simulink model "Project_simulation_v2"  (R2022b)
settings: Solver=VariableStepAuto  StartTime=0.0  StopTime=15  RelTol=1e-3
libraries: spsDiodeLib x7, simulink x4, spsVoltageMeasurementLib x4, spsACVoltageSourceLib x3, spsCurrentMeasurementLib x3, spsMeanLib x3, spsRMSLib x2, spsDCMachineLib x1, spsDCVoltageSourceLib x1, spsIGBTLib x1, spsSeriesRLCBranchLib x1, sps_lib x1
settings Model: Creator=tunaa  LastModifiedBy=tunaa

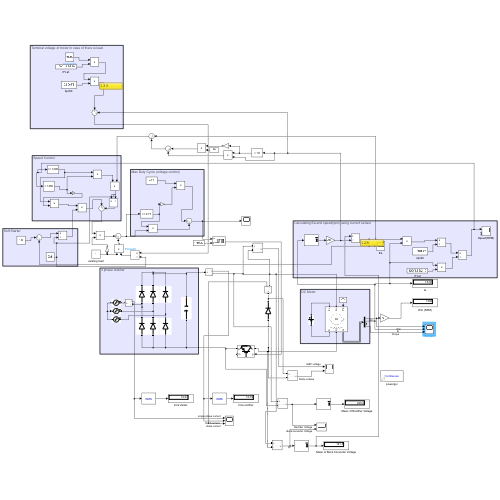
[thumbnail: Simulink's stored preview of the top-level diagram]
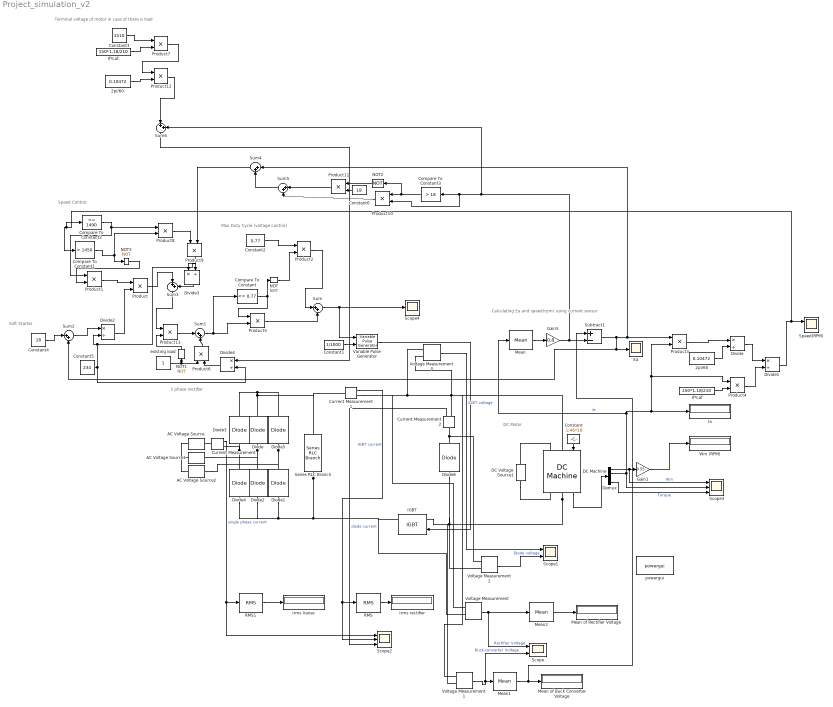
== system Project_simulation_v2 ==
  note: Speed Control
  note: DC Motor
  note: 3 phase rectifier
  note: Max Duty Cycle (voltage control)
  note: Calculating Ea and speed(rpm) using current sensor
  note: Soft Starter
  note: Terminal voltage of motor in case of there is load
  2pi/60 : Constant  Value=0.10472
  2pi/60. : Constant  Value=0.10472
  AC Voltage Source : spsACVoltageSourceLib/AC Voltage Source  Amplitude=136  Phase=0  Frequency=50  SampleTime=0  Measurements=None  BusType=swing  Pref=10e3  Qref=0  Qmin=-inf  Qmax=+inf
  AC Voltage Source1 : spsACVoltageSourceLib/AC Voltage Source  Amplitude=136  Phase=-120  Frequency=50  SampleTime=0  Measurements=None  BusType=swing  Pref=10e3  Qref=0  Qmin=-inf  Qmax=+inf
  AC Voltage Source2 : spsACVoltageSourceLib/AC Voltage Source  Amplitude=136  Phase=-240  Frequency=50  SampleTime=0  Measurements=None  BusType=swing  Pref=10e3  Qref=0  Qmin=-inf  Qmax=+inf
  Compare To Constant : simulink/Logic and Bit Operations/Compare To Constant  relop=<=  const=0.77  OutDataTypeStr=boolean
  Compare To Constant1 : simulink/Logic and Bit Operations/Compare To Constant  relop=>  const=1450  OutDataTypeStr=boolean
  Compare To Constant2 : simulink/Logic and Bit Operations/Compare To Constant  relop=<=  const=1490  OutDataTypeStr=boolean
  Compare To Constant3 : simulink/Logic and Bit Operations/Compare To Constant  relop=>  const=18  OutDataTypeStr=boolean
  Constant : Constant  Value=1.46*10
  Constant1 : Constant  Value=1/1000
  Constant2 : Constant  Value=0.77
  Constant3 : Constant  Value=1510
  Constant4 : Constant  Value=18
  Constant5 : Constant  Value=234
  Constant6 : Constant  Value=18
  Current Measurement : spsCurrentMeasurementLib/Current Measurement  PhasorSimulation=off  OutputType=Complex  PSBequivalent=0
  Current Measurement1 : spsCurrentMeasurementLib/Current Measurement  PhasorSimulation=off  OutputType=Complex  PSBequivalent=0
  Current Measurement2 : spsCurrentMeasurementLib/Current Measurement  PhasorSimulation=off  OutputType=Complex  PSBequivalent=0
  DC Machine : spsDCMachineLib/DC Machine  PresetModel=No  MechanicalLoad=Torque TL  FieldType=Wound  ShowDetailedParameters=on  MeasurementBus=off  RLa="[ 0.8  0.0125]"  RLf="[ 210  23]"  Laf=1.18  MachineConstant=Torque constant (N.m/A)  Ke=1.8  Kt=1.8  J=1  Bm=0  Tf=0  w0=157  Ifinit=0.714285714285714  TsPowergui=0  TsBlock=-1
  DC Voltage Source1 : spsDCVoltageSourceLib/DC Voltage Source  Amplitude=150  Measurements=None
  Demux : Demux
  Diode{,1..6} (7 alike) : spsDiodeLib/Diode  Ron=0.001  Lon=0  Vf=0.8  IC=0  UseSnubber=0  Rs=0  Cs=0  Measurements=off
  Divide{,1..4} (5 alike) : Product  Inputs=*/
  Ea : Scope
  Gain1 : Gain  Gain=9.55
  Gain5 : Gain  Gain=0.8
  IGBT : spsIGBTLib/IGBT  Ron=0.001  Lon=0  Vf=1  Tf=1e-6  Tt=2e-6  IC=0  Rs=1e5  Cs=inf  Measurements=on
  Ia : Display
  If*Laf : Constant  Value=150*1.18/210
  If*Laf. : Constant  Value=150*1.18/210
  Irms Variac : Display
  Irms rectifier : Display
  Mean : spsMeanLib/Mean  Freq=1000  Vinit=0  Ts=0
  Mean of Buck Converter Voltage : Display
  Mean of Rectifier Voltage : Display
  Mean1 : spsMeanLib/Mean  Freq=50  Vinit=0  Ts=0
  Mean2 : spsMeanLib/Mean  Freq=50  Vinit=0  Ts=0
  NOT{,1..3} (4 alike) : Logic  Operator=NOT  IconShape=distinctive  AllPortsSameDT=off  OutDataTypeStr=boolean
  Product{,1..13} (14 alike) : Product
  RMS : spsRMSLib/RMS  TrueRMS=on  Freq=50  RMSInit=0  Ts=0
  RMS1 : spsRMSLib/RMS  TrueRMS=on  Freq=50  RMSInit=0  Ts=0
  Scope : Scope  NumInputPorts=2
  Scope1 : Scope  NumInputPorts=2
  Scope2 : Scope  NumInputPorts=3
  Scope3 : Scope  NumInputPorts=3
  Scope4 : Scope
  Series RLC Branch : spsSeriesRLCBranchLib/Series RLC Branch  LConnTagsString=__new0  RConnTagsString=__new0  BranchType=C  Resistance=1  Inductance=1e-3  SetiL0=off  InitialCurrent=0  Capacitance=2*470e-6  Setx0=off  InitialVoltage=0  Measurements=None
  Speed(RPM) : Scope  NumInputPorts=2
  Subtract1 : Sum  Inputs=+-
  Sum{,1..6} (7 alike) : Sum  Inputs=|++
  Variable Pulse Generator : VariablePulseGenerator  AllowZeroPulseWidth=on  SampleTime=0.1
  Voltage Measurement{,1..3} (4 alike) : spsVoltageMeasurementLib/Voltage Measurement  PhasorSimulation=off  OutputType=Complex  PSBequivalent=0
  Wm (RPM) : Display
  existing load : Constant
  powergui : sps_lib/powergui  Priority=1  SimulationMode=Continuous  SampleTime=50e-6  frequency=60  Iterations=50  frequencyindice=50  Pbase=100e6  ErrMax=1e-4  UnitsV=kV  UnitsW=MW  buscounter=0  FunctionMessages=off  echomessages=off  EnableUseOfTLC=off  CurrentSourceSwitches=off  DisableSnubberDevices=off  DisableRonSwitches=off  DisableVfSwitches=off  DisplayEquations=off  AutomaticDiscreteSolvers=off  SolverType=Tustin/Backward Euler (TBE)  Interpol=off  ExternalGateDelay=off  methode=off  Ts=100  x0status=blocks  SPID=on  SwTol=0  HookPort=off  NonlinearTolerance=1e-4  nMaxIteration=100  ContinueOnMaxIteration=off  RestoreLinks=warning  ResistiveCurrentMeasurement=off  Frange=[0:2:500]  Ylog=off  Xlog=on  ShowGrid=off  save=off  variable=ZData  structure=0  ZoomFFT=off  StartTime=0.0  cycles=1  DisplayStyle=1  fundamental=60  FreqAxis=off  MaxFrequency=1000  frequencyindicesteady=1  RmsSteady=1  display=off
  wires:
  Current Measurement2/1 -> Scope2/3  "diode current"
  Subtract1/1 -> Sum2/2, Ea/1, Sum4/1, Product3/1
  Gain1/1 -> Wm (RPM)/1
  Demux/1 -> Scope3/1, Gain1/1  "Wm"
  Voltage Measurement3/1 -> Scope1/1  "IGBT voltage"
  Constant/1 -> DC Machine/1
  Constant2/1 -> Product2/1
  Demux/4 -> Scope3/3  "Torque"
  Product4/1 -> Divide1/2
  Constant5/1 -> Divide3/2, Divide2/2, Divide4/2
  Product2/1 -> Sum/1
  Constant4/1 -> Sum2/1
  Divide2/1 -> Product/2
  Current Measurement/1 -> Scope2/1, RMS1/1  "single phase current"
  Sum/1 -> Variable Pulse Generator/1, Scope4/1
  Product1/1 -> Product/1
  Compare To Constant/1 -> Product5/1, NOT/1
  NOT/1 -> Product2/2
  Divide/1 -> Divide1/1
  2pi/60/1 -> Divide/2
  Product5/1 -> Sum/2
  Product3/1 -> Divide/1
  Variable Pulse Generator/1 -> IGBT/1
  RMS/1 -> Irms rectifier/1
  Current Measurement1/1 -> Scope2/2, RMS/1  "IGBT current"
  Demux/2 -> Mean/1, Product4/1, Product3/2, Ia/1, Scope3/2  "Ia"
  RMS1/1 -> Irms Variac/1
  Sum2/1 -> Divide2/1
  Mean1/1 -> Subtract1/1, Mean of Buck Converter Voltage/1
  Voltage Measurement1/1 -> Scope/2, Mean1/1  "Buck-converter Voltage"
  Voltage Measurement/1 -> Scope/1, Mean2/1  "Rectifier Voltage"
  Constant1/1 -> Variable Pulse Generator/2
  DC Machine/1 -> Demux/1
  If*Laf/1 -> Product4/2
  Gain5/1 -> Sum6/2, Product10/2, Compare To Constant3/1, Subtract1/2
  Mean2/1 -> Mean of Rectifier Voltage/1
  Voltage Measurement2/1 -> Scope1/2  "Diode voltage"
  Mean/1 -> Gain5/1
  Compare To Constant1/1 -> NOT3/1, Product8/2
  NOT3/1 -> Product1/2
  Compare To Constant2/1 -> Product1/1, Product8/1
  Product8/1 -> Product9/1
  Product/1 -> Sum3/1
  Compare To Constant3/1 -> NOT2/1, Product10/1
  NOT2/1 -> Product11/1
  Constant6/1 -> Product11/2
  Product10/1 -> Sum5/2
  Product11/1 -> Sum5/1
  Sum5/1 -> Sum4/2
  Product9/1 -> Divide3/1
  Divide3/1 -> Sum3/2
  Divide1/1 -> Compare To Constant1/1, Compare To Constant2/1, Speed(RPM)/1
  Sum4/1 -> Product9/2
  If*Laf./1 -> Product7/2
  2pi/60./1 -> Product12/2
  Product7/1 -> Product12/1
  Product12/1 -> Sum6/1
  existing load/1 -> NOT1/1, Product6/1
  Product6/1 -> Sum1/2
  Sum3/1 -> Product13/1
  NOT1/1 -> Product13/2
  Product13/1 -> Sum1/1
  Sum1/1 -> Compare To Constant/1, Product5/2
  Sum6/1 -> Divide4/1
  Divide4/1 -> Product6/2
  Constant3/1 -> Product7/1
  connections:
  DC Machine/RConn1 -- Voltage Measurement2/LConn2 -- Diode6/LConn1 -- IGBT/LConn1 -- Voltage Measurement1/LConn2
  Voltage Measurement3/LConn1 -- Current Measurement1/RConn1 -- Voltage Measurement/LConn1 -- DC Machine/LConn1 -- Voltage Measurement1/LConn1 -- Voltage Measurement3/LConn2 -- Current Measurement2/RConn1
  Diode6/RConn1 -- Voltage Measurement2/LConn1 -- Current Measurement2/LConn1
  Diode3/RConn1 -- Series RLC Branch/LConn1 -- Current Measurement1/LConn1 -- Diode/RConn1 -- Diode5/RConn1
  Series RLC Branch/RConn1 -- Diode4/LConn1 -- Diode2/LConn1 -- Diode1/LConn1 -- IGBT/RConn1 -- Voltage Measurement/LConn2
  Diode5/LConn1 -- AC Voltage Source2/RConn1 -- Diode1/RConn1
  Diode3/LConn1 -- Diode4/RConn1 -- Current Measurement/RConn1
  AC Voltage Source1/LConn1 -- AC Voltage Source/LConn1 -- AC Voltage Source2/LConn1
  Diode/LConn1 -- AC Voltage Source1/RConn1 -- Diode2/RConn1
  Current Measurement/LConn1 -- AC Voltage Source/RConn1
  DC Voltage Source1/RConn1 -- DC Machine/LConn2
  DC Voltage Source1/LConn1 -- DC Machine/RConn2
